simulink model "DA40_Flight_Model"  (R2023a)
settings: Solver=FixedStepAuto  StartTime=DCAM.startTime  StopTime=DCAM.endTime  FixedStep=DCAM.timeStep  RelTol=1e-3
undefined symbols (not defined in the file or in its folder): DCAM, Earth, WGS84
libraries: simulink x27, slpidlib x15, simulink_extras x6, sharedtransform x4, aerolibtransform2 x4, aerolibatmos2 x3, uavalgslib x2, aerolibwind2 x1
(part 1 of 6)
settings Model: Creator=izc0018  LastModifiedBy=noahm
settings DebuggingCC: AlgebraicLoopMsg=none  UnconnectedInputMsg=warning  UnconnectedOutputMsg=warning  UnconnectedLineMsg=warning
settings HardwareCC: ProdBitPerLong=64  ProdLargestAtomicFloat=None  ProdHWDeviceType=AMD->Athlon 64
settings ModelReferenceCC: EnableRefExpFcnMdlSchedulingChecks=on  ModelReferenceMinAlgLoopOccurrences=on
settings RTWCC: DLArmComputeVersion=19.05

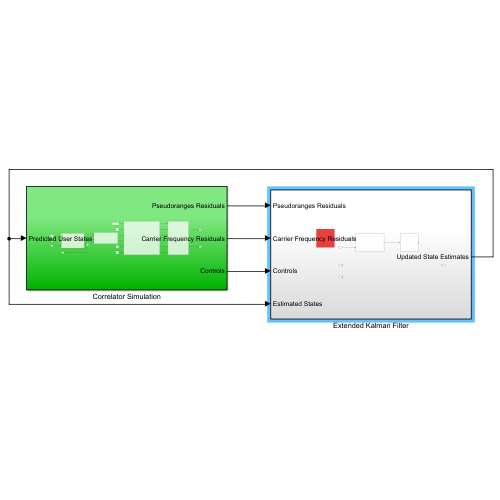
[thumbnail: Simulink's stored preview of the top-level diagram]
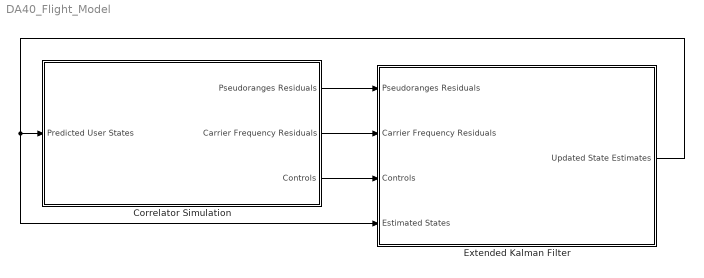
== system DA40_Flight_Model ==
  Correlator Simulation : Subsystem
  Extended Kalman Filter : Subsystem
  wires:
  Extended Kalman Filter/1(Updated State Estimates) -> Extended Kalman Filter/4(Estimated States), Correlator Simulation/1(Predicted User States)
  Correlator Simulation/1(Pseudoranges Residuals) -> Extended Kalman Filter/1(Pseudoranges Residuals)
  Correlator Simulation/2(Carrier Frequency Residuals) -> Extended Kalman Filter/2(Carrier Frequency Residuals)
  Correlator Simulation/3(Controls) -> Extended Kalman Filter/3(Controls)

== system DA40_Flight_Model/Correlator Simulation ==
  Predicted User States : Inport
  Band-Limited White Noise : simulink/Sources/Band-Limited White Noise  Cov=1  Ts=1/50  seed=DCAM.currentSeed
  Clock : Clock
  Constant : Constant  Value=0.5
  Constant1 : Constant  Value=1/50
  Constant2 : Constant  Value=10^(45/10)
  Constant3 : Constant  Value=0
  MATLAB Function : MATLAB Function  TreatAsAtomicUnit=on
  MATLAB Function1 : MATLAB Function  TreatAsAtomicUnit=on
  Subsystem : Subsystem
  Subsystem1 : Subsystem
  Terminator : Terminator
  Pseudoranges Residuals : Outport
  Carrier Frequency Residuals : Outport  Port=2
  Controls : Outport  Port=3
  wires:
  Constant/1 -> MATLAB Function/5(offset)
  Constant1/1 -> MATLAB Function/2(pdiTime)
  Band-Limited White Noise/1 -> MATLAB Function/6(whiteNoise)
  Constant2/1 -> MATLAB Function/1(cno)
  Subsystem/1(carrFreqError) -> MATLAB Function/3(carrFreqError)
  Subsystem/2(codeFreqError) -> MATLAB Function/4(codePhaseError)
  Constant3/1 -> Subsystem1/1(time)
  Clock/1 -> Subsystem1/2(time1)
  Subsystem1/1(MeasuredCarrierFrequency) -> Subsystem/1(measuredCarrierFrequency)
  Subsystem1/2(MeasuredCodeFrequency) -> Subsystem/2(measuredCodeFrequency)
  Subsystem1/6(Controls) -> Controls/1
  Predicted User States/1 -> Subsystem1/3(Predicted User States)
  Subsystem1/4(EstimatedCodeFrequency) -> Subsystem/4(estimatedCodeFrequency)
  Subsystem1/3(EstimatedCarrierFrequency) -> Subsystem/3(estimatedCarrierFrequency)
  MATLAB Function/6(QL) -> MATLAB Function1/6(QL)
  MATLAB Function/5(IL) -> MATLAB Function1/5(IL)
  MATLAB Function/4(QP) -> MATLAB Function1/4(QP)
  MATLAB Function/3(IP) -> MATLAB Function1/3(IP)
  MATLAB Function/2(QE) -> MATLAB Function1/2(QE)
  MATLAB Function/1(IE) -> MATLAB Function1/1(IE)
  MATLAB Function1/2(codeFreqResiduals) -> Pseudoranges Residuals/1
  MATLAB Function1/1(carrierFreqResiduals) -> Carrier Frequency Residuals/1
  Subsystem1/5(Measured Pseudoranges) -> Terminator/1

== system DA40_Flight_Model/Extended Kalman Filter ==
  Pseudoranges Residuals : Inport
  Carrier Frequency Residuals : Inport  Port=2
  Controls : Inport  Port=3
  Estimated States : Inport  Port=4
  Body To ECEF : Subsystem
  ECEF to BODY : Subsystem
  Noise Model : Subsystem
  Updated State Estimates : Outport
  wires:
  Noise Model/1(Predicted States) -> Body To ECEF/1(Predicted States)
  Controls/1 -> Noise Model/2(Controls)
  ECEF to BODY/1(ECEF States) -> Noise Model/1(Estimated States)
  Estimated States/1 -> ECEF to BODY/1(Estimated States)

== system DA40_Flight_Model/Correlator Simulation/Subsystem ==
  measuredCarrierFrequency : Inport
  measuredCodeFrequency : Inport  Port=2
  estimatedCarrierFrequency : Inport  Port=3
  estimatedCodeFrequency : Inport  Port=4
  MATLAB Function1 : MATLAB Function  TreatAsAtomicUnit=on
  MATLAB Function2 : MATLAB Function  TreatAsAtomicUnit=on
  carrFreqError : Outport
  codeFreqError : Outport  Port=2
  wires:
  measuredCarrierFrequency/1 -> MATLAB Function1/1(measuredCarrierFrequency)
  estimatedCarrierFrequency/1 -> MATLAB Function1/2(estimatedCarrierFrequency)
  MATLAB Function1/1(carrFreqError) -> carrFreqError/1
  estimatedCodeFrequency/1 -> MATLAB Function2/2(estimatedCodeFrequency)
  MATLAB Function2/1(codeFreqError) -> codeFreqError/1
  measuredCodeFrequency/1 -> MATLAB Function2/1(measuredCodeFrequency)

== system DA40_Flight_Model/Correlator Simulation/Subsystem1 ==
  time : Inport
  time1 : Inport  Port=2
  Predicted User States : Inport  Port=3
  Generating GPS and Satellite Measurements : Subsystem
  Generating GPS and Satellite Measurements1 : Subsystem
  Subsystem2 : Subsystem
  MeasuredCarrierFrequency : Outport
  MeasuredCodeFrequency : Outport  Port=2
  EstimatedCarrierFrequency : Outport  Port=3
  EstimatedCodeFrequency : Outport  Port=4
  Measured Pseudoranges : Outport  Port=5
  Controls : Outport  Port=6
  wires:
  Generating GPS and Satellite Measurements/2(Satellite States) -> Subsystem2/4(Satellite States)
  Subsystem2/1(MeasuredCarrierFrequency) -> MeasuredCarrierFrequency/1
  Generating GPS and Satellite Measurements/3(Controls) -> Controls/1
  Generating GPS and Satellite Measurements/1(GPS User States) -> Subsystem2/3(GPS User States)
  Generating GPS and Satellite Measurements1/1(GPS User States) -> Subsystem2/1(Initial GPS User States)
  Generating GPS and Satellite Measurements1/2(Satellite States) -> Subsystem2/2(Initial Satellite States)
  Subsystem2/2(MeasuredCodeFrequency) -> MeasuredCodeFrequency/1
  time1/1 -> Generating GPS and Satellite Measurements/1(time)
  time/1 -> Generating GPS and Satellite Measurements1/1(time)
  Subsystem2/3(Measured Pseudoranges) -> Measured Pseudoranges/1
  Predicted User States/1 -> Subsystem2/5(Predicted User States)
  Subsystem2/4(EstimatedCarrierFrequency) -> EstimatedCarrierFrequency/1
  Subsystem2/5(EstimatedCodeFrequency) -> EstimatedCodeFrequency/1

== system DA40_Flight_Model/Extended Kalman Filter/Body To ECEF ==
  Predicted States : Inport
  Bus Creator : BusCreator  Inputs=8
  Bus Selector : BusSelector  OutputSignals=psi,theta,phi
  Bus Selector1 : BusSelector  OutputSignals=x,y,z
  Bus Selector2 : BusSelector  OutputSignals=x,y,z,u,v,w
  Constant : Constant  Value=0
  Constant1 : Constant  Value=89.0
  Constant2 : Constant  Value=0
  Direction Cosine Matrix ECEF to NED : aerolibtransform2/Direction Cosine Matrix ECEF to NED
  Flat Earth to LLA : aerolibtransform2/Flat Earth to LLA  units=Metric (MKS)  ptype=Earth (WGS84)  F=1/298.257223563  R=6378137  refPosPort=off  LL0=DCAM.FVDM.refLL  psi=0
  MATLAB Function : MATLAB Function  TreatAsAtomicUnit=on
  MATLAB Function1 : MATLAB Function  TreatAsAtomicUnit=on
  Rotation Angles to Direction Cosine Matrix : sharedtransform/Rotation Angles to Direction Cosine Matrix  rotationOrder=ZYX  aMode=aMode
  Terminator : Terminator
  Transpose : Math  Operator=transpose
  Vector Concatenate{,1..3} (4 alike) : Concatenate  NumInputs=3
  ECEF States : Outport
  wires:
  Predicted States/1 -> Bus Selector2/1, Bus Selector1/1, Bus Selector/1
  Bus Selector/1 -> Vector Concatenate/1  "<psi>"
  Bus Selector/2 -> Vector Concatenate/2  "<theta>"
  Bus Selector/3 -> Vector Concatenate/3  "<phi>"
  Vector Concatenate/1 -> Rotation Angles to Direction Cosine Matrix/1
  Flat Earth to LLA/1 -> Direction Cosine Matrix ECEF to NED/1
  Flat Earth to LLA/2 -> Terminator/1
  Constant/1 -> Flat Earth to LLA/2
  Vector Concatenate1/1 -> Flat Earth to LLA/1
  Bus Selector1/1 -> Vector Concatenate1/1  "<x>"
  Bus Selector1/2 -> Vector Concatenate1/2  "<y>"
  Bus Selector1/3 -> Vector Concatenate1/3  "<z>"
  Direction Cosine Matrix ECEF to NED/1 -> Transpose/1
  Transpose/1 -> MATLAB Function/2(DCM_NE)  "NED TO ECEF"
  Rotation Angles to Direction Cosine Matrix/1 -> MATLAB Function/1(DCM_BN)  "BODY TO NED"
  MATLAB Function/1(DCM_BE) -> MATLAB Function1/5(DCM_BE)
  MATLAB Function1/8(clkBias) -> Bus Creator/8
  MATLAB Function1/7(clk) -> Bus Creator/7
  MATLAB Function1/6(w) -> Bus Creator/6
  MATLAB Function1/5(v) -> Bus Creator/5
  MATLAB Function1/4(u) -> Bus Creator/4
  MATLAB Function1/3(z) -> Bus Creator/3
  MATLAB Function1/2(y) -> Bus Creator/2
  MATLAB Function1/1(x) -> Bus Creator/1
  Bus Creator/1 -> ECEF States/1
  Constant1/1 -> MATLAB Function1/4("clkBias ")
  Constant2/1 -> MATLAB Function1/3("clk ")
  Vector Concatenate2/1 -> MATLAB Function1/1(pos)
  Vector Concatenate3/1 -> MATLAB Function1/2(vel)
  Bus Selector2/1 -> Vector Concatenate2/1  "<x>"
  Bus Selector2/2 -> Vector Concatenate2/2  "<y>"
  Bus Selector2/3 -> Vector Concatenate2/3  "<z>"
  Bus Selector2/4 -> Vector Concatenate3/1  "<u>"
  Bus Selector2/5 -> Vector Concatenate3/2  "<v>"
  Bus Selector2/6 -> Vector Concatenate3/3  "<w>"

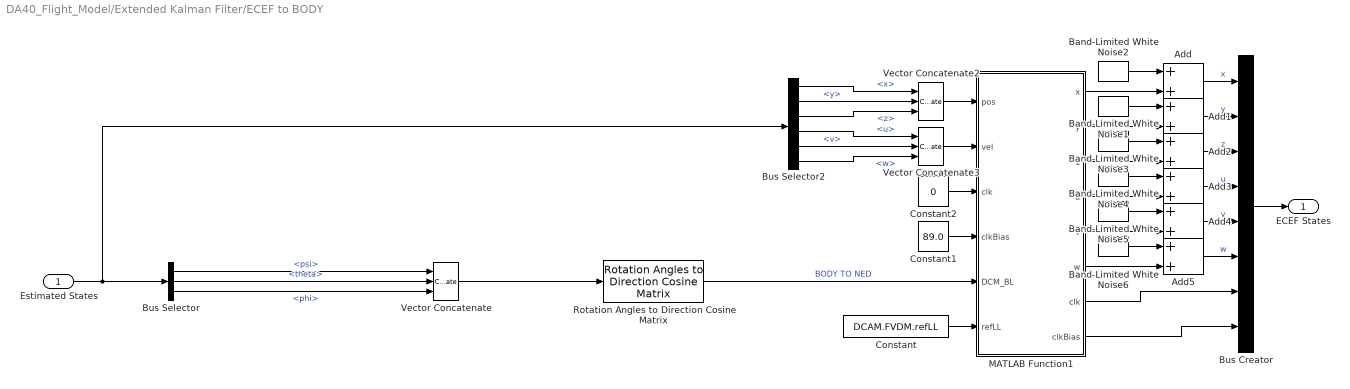
== system DA40_Flight_Model/Extended Kalman Filter/ECEF to BODY ==
  Estimated States : Inport
  Add{,1..5} (6 alike) : Sum
  Band-Limited White Noise1 : simulink/Sources/Band-Limited White Noise  Cov=1.5  Ts=1/50  seed=[23341]
  Band-Limited White Noise2 : simulink/Sources/Band-Limited White Noise  Cov=1.5  Ts=1/50  seed=[23341]
  Band-Limited White Noise3 : simulink/Sources/Band-Limited White Noise  Cov=3  Ts=1/50  seed=[23341]
  Band-Limited White Noise4 : simulink/Sources/Band-Limited White Noise  Cov=0.15  Ts=1/50  seed=[23341]
  Band-Limited White Noise5 : simulink/Sources/Band-Limited White Noise  Cov=0.15  Ts=1/50  seed=[23341]
  Band-Limited White Noise6 : simulink/Sources/Band-Limited White Noise  Cov=0.3  Ts=1/50  seed=[23341]
  Bus Creator : BusCreator  Inputs=8
  Bus Selector : BusSelector  OutputSignals=psi,theta,phi
  Bus Selector2 : BusSelector  OutputSignals=x,y,z,u,v,w
  Constant : Constant  Value=DCAM.FVDM.refLL
  Constant1 : Constant  Value=89.0
  Constant2 : Constant  Value=0
  MATLAB Function1 : MATLAB Function  TreatAsAtomicUnit=on
  Rotation Angles to Direction Cosine Matrix : sharedtransform/Rotation Angles to Direction Cosine Matrix  rotationOrder=ZYX  aMode=aMode
  Vector Concatenate : Concatenate  NumInputs=3
  Vector Concatenate2 : Concatenate  NumInputs=3
  Vector Concatenate3 : Concatenate  NumInputs=3
  ECEF States : Outport
  wires:
  Estimated States/1 -> Bus Selector2/1, Bus Selector/1
  Bus Selector/1 -> Vector Concatenate/1  "<psi>"
  Bus Selector/2 -> Vector Concatenate/2  "<theta>"
  Bus Selector/3 -> Vector Concatenate/3  "<phi>"
  Vector Concatenate/1 -> Rotation Angles to Direction Cosine Matrix/1
  Rotation Angles to Direction Cosine Matrix/1 -> MATLAB Function1/5(DCM_BL)  "BODY TO NED"
  MATLAB Function1/8(clkBias) -> Bus Creator/8
  MATLAB Function1/7(clk) -> Bus Creator/7
  Bus Creator/1 -> ECEF States/1
  Constant1/1 -> MATLAB Function1/4("clkBias ")
  Constant2/1 -> MATLAB Function1/3("clk ")
  Vector Concatenate2/1 -> MATLAB Function1/1(pos)
  Vector Concatenate3/1 -> MATLAB Function1/2(vel)
  Bus Selector2/1 -> Vector Concatenate2/1  "<x>"
  Bus Selector2/2 -> Vector Concatenate2/2  "<y>"
  Bus Selector2/3 -> Vector Concatenate2/3  "<z>"
  Bus Selector2/4 -> Vector Concatenate3/1  "<u>"
  Bus Selector2/5 -> Vector Concatenate3/2  "<v>"
  Bus Selector2/6 -> Vector Concatenate3/3  "<w>"
  Add/1 -> Bus Creator/1  "x"
  MATLAB Function1/1(x) -> Add/2
  Add1/1 -> Bus Creator/2  "y"
  Add2/1 -> Bus Creator/3  "z"
  Add3/1 -> Bus Creator/4  "u"
  Add4/1 -> Bus Creator/5  "v"
  Add5/1 -> Bus Creator/6  "w"
  Band-Limited White Noise1/1 -> Add1/1
  Band-Limited White Noise2/1 -> Add/1
  Band-Limited White Noise3/1 -> Add2/1
  Band-Limited White Noise4/1 -> Add3/1
  Band-Limited White Noise5/1 -> Add4/1
  Band-Limited White Noise6/1 -> Add5/1
  MATLAB Function1/2(y) -> Add1/2
  MATLAB Function1/3(z) -> Add2/2
  MATLAB Function1/4(u) -> Add3/2
  MATLAB Function1/5(v) -> Add4/2
  MATLAB Function1/6(w) -> Add5/2
  Constant/1 -> MATLAB Function1/6(refLL)

== system DA40_Flight_Model/Extended Kalman Filter/Noise Model ==
  Estimated States : Inport
  Controls : Inport  Port=2
  Band-Limited White Noise1 : simulink/Sources/Band-Limited White Noise  Cov=DCAM.FVDM.wind.direction  Ts=DCAM.FVDM.wind.directionTS  seed=DCAM.currentSeed
  Band-Limited White Noise3 : simulink/Sources/Band-Limited White Noise  Cov=DCAM.FVDM.wind.velocity  Ts=DCAM.FVDM.wind.velocityTS  seed=DCAM.currentSeed
  Environment : Subsystem
  Navigation : Subsystem
  Predicted States : Outport
  wires:
  Environment/1(Atmos) -> Navigation/1(Atmosphere)
  Navigation/1(States) -> Predicted States/1
  Band-Limited White Noise3/1 -> Environment/2(Wind Velocity)
  Controls/1 -> Navigation/2(Controls)
  Band-Limited White Noise1/1 -> Environment/3(Wind Direction)
  Estimated States/1 -> Environment/1(States)

== system DA40_Flight_Model/Correlator Simulation/Subsystem1/Generating GPS and Satellite Measurements ==
  time : Inport
  Body To ECEF : Subsystem
  Calculate Satellite Positions : Subsystem
  Truth Model : Subsystem
  GPS User States : Outport
  Satellite States : Outport  Port=2
  Controls : Outport  Port=3
  wires:
  time/1 -> Calculate Satellite Positions/1(time)
  Calculate Satellite Positions/1(Satellite States) -> Satellite States/1
  Truth Model/2(Truth States) -> Body To ECEF/1(Predicted States)
  Body To ECEF/1(ECEF States) -> GPS User States/1
  Truth Model/1(Controls) -> Controls/1

== system DA40_Flight_Model/Correlator Simulation/Subsystem1/Generating GPS and Satellite Measurements1 ==
  time : Inport
  Body To ECEF : Subsystem
  Calculate Satellite Positions : Subsystem
  Truth Model : Subsystem
  GPS User States : Outport
  Satellite States : Outport  Port=2
  wires:
  time/1 -> Calculate Satellite Positions/1(time)
  Calculate Satellite Positions/1(Satellite States) -> Satellite States/1
  Truth Model/1(Truth States) -> Body To ECEF/1(Predicted States)
  Body To ECEF/1(ECEF States) -> GPS User States/1

== system DA40_Flight_Model/Correlator Simulation/Subsystem1/Subsystem2 ==
  Initial GPS User States : Inport
  Initial Satellite States : Inport  Port=2
  GPS User States : Inport  Port=3
  Satellite States : Inport  Port=4
  Predicted User States : Inport  Port=5
  Generating PSR/Carrier Frequency Measurements : Subsystem
  Generating PSR/Carrier Frequency Measurements1 : Subsystem
  Generating PSR/Carrier Frequency Measurements2 : Subsystem
  Subsystem1 : Subsystem
  Subsystem2 : Subsystem
  Subsystem3 : Subsystem
  Subsystem4 : Subsystem
  MeasuredCarrierFrequency : Outport
  MeasuredCodeFrequency : Outport  Port=2
  Measured Pseudoranges : Outport  Port=3
  EstimatedCarrierFrequency : Outport  Port=4
  EstimatedCodeFrequency : Outport  Port=5
  wires:
  Subsystem3/1(sampleVector) -> Subsystem1/1(sampleVector)
  Generating PSR/Carrier Frequency Measurements/2(Measured Doppler) -> Subsystem3/5(doppler)
  Subsystem3/2(carrierChangePerSample) -> Subsystem1/2(carrierChangePerSample)
  Generating PSR/Carrier Frequency Measurements/1(Measured Carrier Frequencies) -> Subsystem3/4(measuredCarrierFrequency)
  Generating PSR/Carrier Frequency Measurements/3(Measured SV Clock Bias) -> Subsystem3/6(svClockBias)
  Subsystem3/3(CarrierFrequency) -> Subsystem1/3(measuredCarrierFrequency)
  GPS User States/1 -> Generating PSR/Carrier Frequency Measurements/1(GPS User States)
  Subsystem3/4(codeChangePerSample) -> Subsystem1/4(codeChangePerSample)
  Subsystem1/1(MeasuredCarrierFrequency) -> MeasuredCarrierFrequency/1
  Subsystem3/5(initialCodePhase) -> Subsystem1/5(initialCodePhase)
  Generating PSR/Carrier Frequency Measurements/4(Measured Pseudoranges) -> Measured Pseudoranges/1
  Satellite States/1 -> Generating PSR/Carrier Frequency Measurements2/1(Satellite States), Generating PSR/Carrier Frequency Measurements/2(Satellite States)
  Subsystem1/2(MeasuredCodeFrequency) -> MeasuredCodeFrequency/1
  Generating PSR/Carrier Frequency Measurements1/4(Initial SV Clock Bias) -> Subsystem3/3(initialSVClockBias)
  Generating PSR/Carrier Frequency Measurements1/3(Initial Doppler) -> Subsystem3/2(initialDoppler)
  Generating PSR/Carrier Frequency Measurements1/2(Initial Carrier Frequencies) -> Subsystem2/1(initialCarrierFrequency), Subsystem3/1(initialCarrierFrequency), Subsystem2/2(initialDoppler), Subsystem2/3(initialSVClockBias)
  Initial Satellite States/1 -> Generating PSR/Carrier Frequency Measurements1/2(Satellite States)
  Initial GPS User States/1 -> Generating PSR/Carrier Frequency Measurements1/1(GPS User States)
  Predicted User States/1 -> Generating PSR/Carrier Frequency Measurements2/2(Predicted User States)
  Generating PSR/Carrier Frequency Measurements2/1(Estimated Carrier Frequencies) -> Subsystem2/4(estimatedCarrierFrequency)
  Generating PSR/Carrier Frequency Measurements2/2(Estimated Doppler) -> Subsystem2/5(doppler)
  Generating PSR/Carrier Frequency Measurements2/3(Estimated SV Clock Bias) -> Subsystem2/6(svClockBias)
  Subsystem2/1(sampleVector) -> Subsystem4/1(sampleVector)
  Subsystem2/2(carrierChangePerSample) -> Subsystem4/2(carrierChangePerSample)
  Subsystem2/3(CarrierFrequency) -> Subsystem4/3(measuredCarrierFrequency)
  Subsystem2/4(codeChangePerSample) -> Subsystem4/4(codeChangePerSample)
  Subsystem2/5(initialCodePhase) -> Subsystem4/5(initialCodePhase)
  Subsystem4/1(EstimatedCarrierFrequency) -> EstimatedCarrierFrequency/1
  Subsystem4/2(EstimatedCodeFrequency) -> EstimatedCodeFrequency/1

== system DA40_Flight_Model/Extended Kalman Filter/Noise Model/Environment ==
  States : Inport
  Wind Velocity : Inport  Port=2
  Wind Direction : Inport  Port=3
  Bus Creator : BusCreator  Inputs=5
  Constant6 : Constant  Value=[3 2 1]
  Gain : Gain  Gain=180/pi
  Gain1 : Gain  Gain=-1
  Horizontal Wind Model : aerolibwind2/Horizontal Wind Model  units=Metric (MKS)  Vw_source=External  Vwind=0  W_source=External  Wdeg=0
  ISA Atmosphere Model : aerolibatmos2/ISA Atmosphere Model  custom=off  g=9.80665  gamma=1.4  R=287.0531  L=0.0065  h_trop=11000  h_strat=20000  rho0=1.225  P0=101325  T0=288.15  h0=0
  MATLAB Function7 : MATLAB Function  TreatAsAtomicUnit=on
  Selector : Selector  InputPortWidth=12  IndexOptions=Index vector (dialog)  Indices=[10 11 12]  OutputSizes=1
  Selector1 : Selector  InputPortWidth=12  IndexOptions=Index vector (dialog)  Indices=[9]  OutputSizes=1
  Atmos : Outport
  wires:
  MATLAB Function7/1(DCM) -> Horizontal Wind Model/1
  States/1 -> Selector/1, Selector1/1
  Selector1/1 -> Gain1/1
  ISA Atmosphere Model/2 -> Bus Creator/2  "Speed of Sound"
  ISA Atmosphere Model/3 -> Bus Creator/3  "Pressure"
  Bus Creator/1 -> Atmos/1
  Selector/1 -> Gain/1
  ISA Atmosphere Model/1 -> Bus Creator/1  "Temperature"
  Gain/1 -> MATLAB Function7/1(RotAngles)
  ISA Atmosphere Model/4 -> Bus Creator/4  "Density"
  Constant6/1 -> MATLAB Function7/2(RotSequence)
  Horizontal Wind Model/1 -> Bus Creator/5  "Wind Vector"
  Gain1/1 -> ISA Atmosphere Model/1
  Wind Velocity/1 -> Horizontal Wind Model/2
  Wind Direction/1 -> Horizontal Wind Model/3

== system DA40_Flight_Model/Extended Kalman Filter/Noise Model/Navigation ==
  Atmosphere : Inport
  Controls : Inport  Port=2
  Constant1 : Constant  Value=DCAM.FVDM.Vehicle.MassProp.Mass
  DA-40 Equations of Motion : Subsystem
  Flight Mechanics and Systems Models : Subsystem
  States : Outport
  wires:
  Flight Mechanics and Systems Models/1(Fb) -> DA-40 Equations of Motion/1(Fb [lb])
  Flight Mechanics and Systems Models/2(Mb) -> DA-40 Equations of Motion/2(Mb [lb-ft])
  Controls/1 -> Flight Mechanics and Systems Models/2(Control Commands)
  Atmosphere/1 -> Flight Mechanics and Systems Models/1(Atmosphere)
  Constant1/1 -> DA-40 Equations of Motion/3(Mass Properties)
  DA-40 Equations of Motion/1(States) -> States/1, Flight Mechanics and Systems Models/3(States)

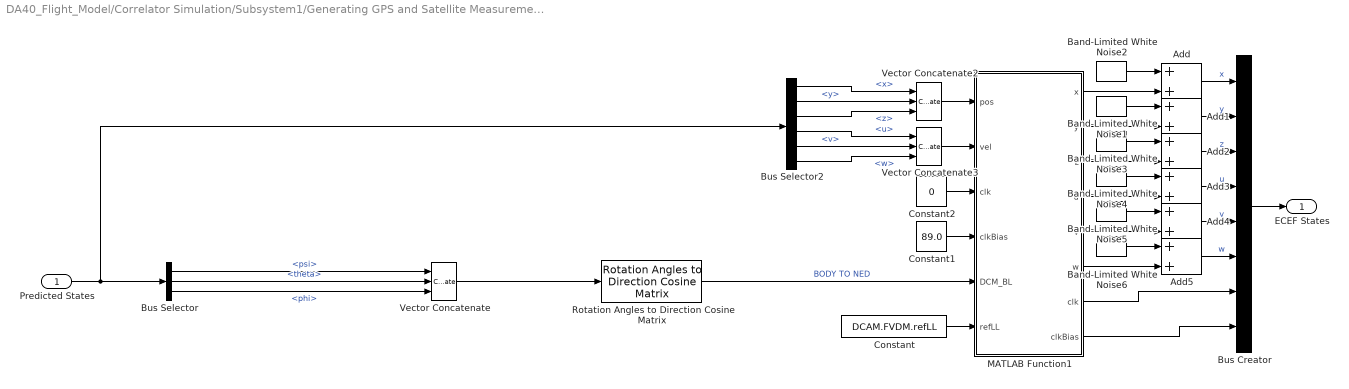
== system DA40_Flight_Model/Correlator Simulation/Subsystem1/Generating GPS and Satellite Measurements/Body To ECEF ==
  Predicted States : Inport
  Add{,1..5} (6 alike) : Sum
  Band-Limited White Noise1 : simulink/Sources/Band-Limited White Noise  Cov=1.5  Ts=1/50  seed=[23341]
  Band-Limited White Noise2 : simulink/Sources/Band-Limited White Noise  Cov=1.5  Ts=1/50  seed=[23341]
  Band-Limited White Noise3 : simulink/Sources/Band-Limited White Noise  Cov=3  Ts=1/50  seed=[23341]
  Band-Limited White Noise4 : simulink/Sources/Band-Limited White Noise  Cov=0.15  Ts=1/50  seed=[23341]
  Band-Limited White Noise5 : simulink/Sources/Band-Limited White Noise  Cov=0.15  Ts=1/50  seed=[23341]
  Band-Limited White Noise6 : simulink/Sources/Band-Limited White Noise  Cov=0.3  Ts=1/50  seed=[23341]
  Bus Creator : BusCreator  Inputs=8
  Bus Selector : BusSelector  OutputSignals=psi,theta,phi
  Bus Selector2 : BusSelector  OutputSignals=x,y,z,u,v,w
  Constant : Constant  Value=DCAM.FVDM.refLL
  Constant1 : Constant  Value=89.0
  Constant2 : Constant  Value=0
  MATLAB Function1 : MATLAB Function  TreatAsAtomicUnit=on
  Rotation Angles to Direction Cosine Matrix : sharedtransform/Rotation Angles to Direction Cosine Matrix  rotationOrder=ZYX  aMode=aMode
  Vector Concatenate : Concatenate  NumInputs=3
  Vector Concatenate2 : Concatenate  NumInputs=3
  Vector Concatenate3 : Concatenate  NumInputs=3
  ECEF States : Outport
  wires:
  Predicted States/1 -> Bus Selector2/1, Bus Selector/1
  Bus Selector/1 -> Vector Concatenate/1  "<psi>"
  Bus Selector/2 -> Vector Concatenate/2  "<theta>"
  Bus Selector/3 -> Vector Concatenate/3  "<phi>"
  Vector Concatenate/1 -> Rotation Angles to Direction Cosine Matrix/1
  Rotation Angles to Direction Cosine Matrix/1 -> MATLAB Function1/5(DCM_BL)  "BODY TO NED"
  MATLAB Function1/8(clkBias) -> Bus Creator/8
  MATLAB Function1/7(clk) -> Bus Creator/7
  Bus Creator/1 -> ECEF States/1
  Constant1/1 -> MATLAB Function1/4("clkBias ")
  Constant2/1 -> MATLAB Function1/3("clk ")
  Vector Concatenate2/1 -> MATLAB Function1/1(pos)
  Vector Concatenate3/1 -> MATLAB Function1/2(vel)
  Bus Selector2/1 -> Vector Concatenate2/1  "<x>"
  Bus Selector2/2 -> Vector Concatenate2/2  "<y>"
  Bus Selector2/3 -> Vector Concatenate2/3  "<z>"
  Bus Selector2/4 -> Vector Concatenate3/1  "<u>"
  Bus Selector2/5 -> Vector Concatenate3/2  "<v>"
  Bus Selector2/6 -> Vector Concatenate3/3  "<w>"
  Add/1 -> Bus Creator/1  "x"
  MATLAB Function1/1(x) -> Add/2
  Add1/1 -> Bus Creator/2  "y"
  Add2/1 -> Bus Creator/3  "z"
  Add3/1 -> Bus Creator/4  "u"
  Add4/1 -> Bus Creator/5  "v"
  Add5/1 -> Bus Creator/6  "w"
  Band-Limited White Noise1/1 -> Add1/1
  Band-Limited White Noise2/1 -> Add/1
  Band-Limited White Noise3/1 -> Add2/1
  Band-Limited White Noise4/1 -> Add3/1
  Band-Limited White Noise5/1 -> Add4/1
  Band-Limited White Noise6/1 -> Add5/1
  MATLAB Function1/2(y) -> Add1/2
  MATLAB Function1/3(z) -> Add2/2
  MATLAB Function1/4(u) -> Add3/2
  MATLAB Function1/5(v) -> Add4/2
  MATLAB Function1/6(w) -> Add5/2
  Constant/1 -> MATLAB Function1/6(refLL)

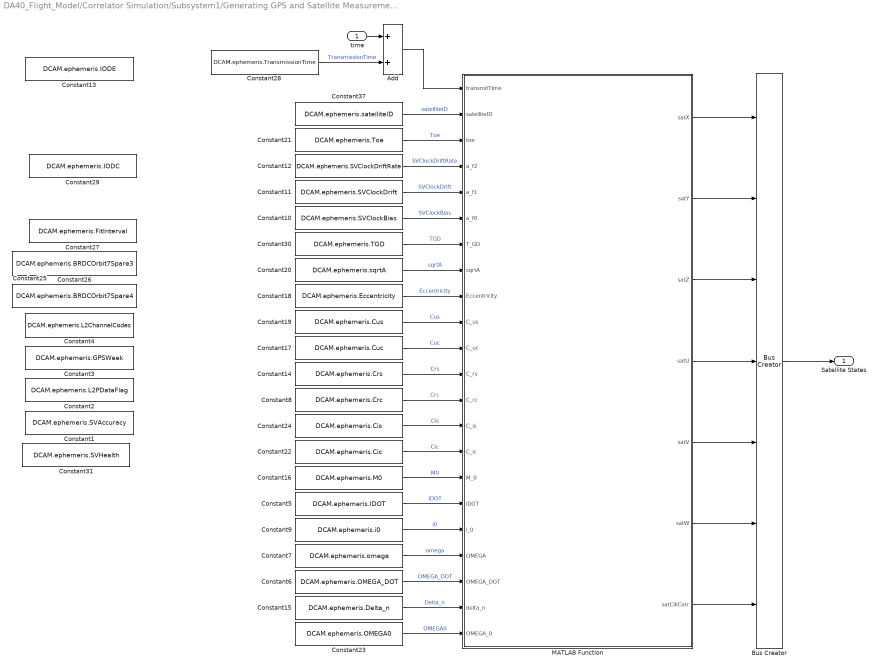
== system DA40_Flight_Model/Correlator Simulation/Subsystem1/Generating GPS and Satellite Measurements/Calculate Satellite Positions ==
  time : Inport
  Add : Sum
  Bus Creator : BusCreator  Inputs=7
  Constant1 : Constant  Value=DCAM.ephemeris.SVAccuracy
  Constant10 : Constant  Value=DCAM.ephemeris.SVClockBias
  Constant11 : Constant  Value=DCAM.ephemeris.SVClockDrift
  Constant12 : Constant  Value=DCAM.ephemeris.SVClockDriftRate
  Constant13 : Constant  Value=DCAM.ephemeris.IODE
  Constant14 : Constant  Value=DCAM.ephemeris.Crs
  Constant15 : Constant  Value=DCAM.ephemeris.Delta_n
  Constant16 : Constant  Value=DCAM.ephemeris.M0
  Constant17 : Constant  Value=DCAM.ephemeris.Cuc
  Constant18 : Constant  Value=DCAM.ephemeris.Eccentricity
  Constant19 : Constant  Value=DCAM.ephemeris.Cus
  Constant2 : Constant  Value=DCAM.ephemeris.L2PDataFlag
  Constant20 : Constant  Value=DCAM.ephemeris.sqrtA
  Constant21 : Constant  Value=DCAM.ephemeris.Toe
  Constant22 : Constant  Value=DCAM.ephemeris.Cic
  Constant23 : Constant  Value=DCAM.ephemeris.OMEGA0
  Constant24 : Constant  Value=DCAM.ephemeris.Cis
  Constant25 : Constant  Value=DCAM.ephemeris.BRDCOrbit7Spare4
  Constant26 : Constant  Value=DCAM.ephemeris.BRDCOrbit7Spare3
  Constant27 : Constant  Value=DCAM.ephemeris.FitInterval
  Constant28 : Constant  Value=DCAM.ephemeris.TransmissionTime
  Constant29 : Constant  Value=DCAM.ephemeris.IODC
  Constant3 : Constant  Value=DCAM.ephemeris.GPSWeek
  Constant30 : Constant  Value=DCAM.ephemeris.TGD
  Constant31 : Constant  Value=DCAM.ephemeris.SVHealth
  Constant37 : Constant  Value=DCAM.ephemeris.satelliteID
  Constant4 : Constant  Value=DCAM.ephemeris.L2ChannelCodes
  Constant5 : Constant  Value=DCAM.ephemeris.IDOT
  Constant6 : Constant  Value=DCAM.ephemeris.OMEGA_DOT
  Constant7 : Constant  Value=DCAM.ephemeris.omega
  Constant8 : Constant  Value=DCAM.ephemeris.Crc
  Constant9 : Constant  Value=DCAM.ephemeris.i0
  MATLAB Function : MATLAB Function  TreatAsAtomicUnit=on
  Satellite States : Outport
  wires:
  Bus Creator/1 -> Satellite States/1
  MATLAB Function/7(satClkCorr) -> Bus Creator/7
  MATLAB Function/6(satW) -> Bus Creator/6
  MATLAB Function/5(satV) -> Bus Creator/5
  MATLAB Function/4(satU) -> Bus Creator/4
  MATLAB Function/3(satZ) -> Bus Creator/3
  MATLAB Function/2(satY) -> Bus Creator/2
  MATLAB Function/1(satX) -> Bus Creator/1
  Constant37/1 -> MATLAB Function/2(satelliteID)  "satelliteID"
  Constant21/1 -> MATLAB Function/3(toe)  "Toe"
  Constant12/1 -> MATLAB Function/4(a_f2)  "SVClockDriftRate"
  Constant11/1 -> MATLAB Function/5(a_f1)  "SVClockDrift"
  Constant10/1 -> MATLAB Function/6(a_f0)  "SVClockBias"
  Constant30/1 -> MATLAB Function/7(T_GD)  "TGD"
  Constant20/1 -> MATLAB Function/8(sqrtA)  "sqrtA"
  Constant18/1 -> MATLAB Function/9(Eccentricity)  "Eccentricity"
  Constant19/1 -> MATLAB Function/10(C_us)  "Cus"
  Constant17/1 -> MATLAB Function/11(C_uc)  "Cuc"
  Constant8/1 -> MATLAB Function/13(C_rc)  "Crc"
  Constant14/1 -> MATLAB Function/12(C_rs)  "Crs"
  Constant24/1 -> MATLAB Function/14(C_is)  "Cis"
  Constant22/1 -> MATLAB Function/15(C_ic)  "Cic"
  Constant16/1 -> MATLAB Function/16(M_0)  "M0"
  Constant5/1 -> MATLAB Function/17(iDOT)  "IDOT"
  Constant9/1 -> MATLAB Function/18(i_0)  "i0"
  Constant7/1 -> MATLAB Function/19(OMEGA)  "omega"
  Constant6/1 -> MATLAB Function/20(OMEGA_DOT)  "OMEGA_DOT"
  Add/1 -> MATLAB Function/1(transmitTime)
  time/1 -> Add/1
  Constant28/1 -> Add/2  "TransmissionTime"
  Constant15/1 -> MATLAB Function/21(delta_n)  "Delta_n"
  Constant23/1 -> MATLAB Function/22(OMEGA_0)  "OMEGA0"

== system DA40_Flight_Model/Correlator Simulation/Subsystem1/Generating GPS and Satellite Measurements/Truth Model ==
  Control : Subsystem
  Environment : Subsystem
  Guidance : Subsystem
  Navigation1 : Subsystem
  Controls : Outport
  Truth States : Outport  Port=2
  wires:
  Control/1(Controls) -> Navigation1/2(Controls), Controls/1
  Guidance/1(Commands) -> Control/1(Commands)
  Guidance/2(States Out) -> Control/2(States)
  Guidance/3(Atmos) -> Control/3(Atmos)
  Environment/1(States Out) -> Guidance/1(States)
  Environment/2(Atmos) -> Guidance/2(Atmosphere)
  Control/3(LLA) -> Environment/2(LLA)
  Control/2(Atmosphere) -> Navigation1/1(Atmosphere)
  Navigation1/1(States) -> Truth States/1, Environment/1(States)

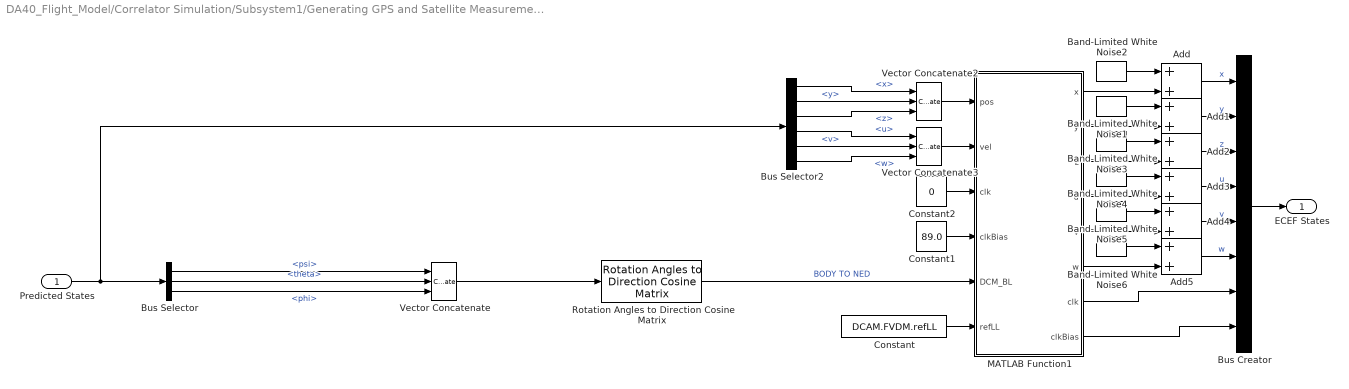
== system DA40_Flight_Model/Correlator Simulation/Subsystem1/Generating GPS and Satellite Measurements1/Body To ECEF ==
  Predicted States : Inport
  Add{,1..5} (6 alike) : Sum
  Band-Limited White Noise1 : simulink/Sources/Band-Limited White Noise  Cov=1.5  Ts=1/50  seed=[23341]
  Band-Limited White Noise2 : simulink/Sources/Band-Limited White Noise  Cov=1.5  Ts=1/50  seed=[23341]
  Band-Limited White Noise3 : simulink/Sources/Band-Limited White Noise  Cov=3  Ts=1/50  seed=[23341]
  Band-Limited White Noise4 : simulink/Sources/Band-Limited White Noise  Cov=0.15  Ts=1/50  seed=[23341]
  Band-Limited White Noise5 : simulink/Sources/Band-Limited White Noise  Cov=0.15  Ts=1/50  seed=[23341]
  Band-Limited White Noise6 : simulink/Sources/Band-Limited White Noise  Cov=0.3  Ts=1/50  seed=[23341]
  Bus Creator : BusCreator  Inputs=8
  Bus Selector : BusSelector  OutputSignals=psi,theta,phi
  Bus Selector2 : BusSelector  OutputSignals=x,y,z,u,v,w
  Constant : Constant  Value=DCAM.FVDM.refLL
  Constant1 : Constant  Value=89.0
  Constant2 : Constant  Value=0
  MATLAB Function1 : MATLAB Function  TreatAsAtomicUnit=on
  Rotation Angles to Direction Cosine Matrix : sharedtransform/Rotation Angles to Direction Cosine Matrix  rotationOrder=ZYX  aMode=aMode
  Vector Concatenate : Concatenate  NumInputs=3
  Vector Concatenate2 : Concatenate  NumInputs=3
  Vector Concatenate3 : Concatenate  NumInputs=3
  ECEF States : Outport
  wires:
  Predicted States/1 -> Bus Selector2/1, Bus Selector/1
  Bus Selector/1 -> Vector Concatenate/1  "<psi>"
  Bus Selector/2 -> Vector Concatenate/2  "<theta>"
  Bus Selector/3 -> Vector Concatenate/3  "<phi>"
  Vector Concatenate/1 -> Rotation Angles to Direction Cosine Matrix/1
  Rotation Angles to Direction Cosine Matrix/1 -> MATLAB Function1/5(DCM_BL)  "BODY TO NED"
  MATLAB Function1/8(clkBias) -> Bus Creator/8
  MATLAB Function1/7(clk) -> Bus Creator/7
  Bus Creator/1 -> ECEF States/1
  Constant1/1 -> MATLAB Function1/4("clkBias ")
  Constant2/1 -> MATLAB Function1/3("clk ")
  Vector Concatenate2/1 -> MATLAB Function1/1(pos)
  Vector Concatenate3/1 -> MATLAB Function1/2(vel)
  Bus Selector2/1 -> Vector Concatenate2/1  "<x>"
  Bus Selector2/2 -> Vector Concatenate2/2  "<y>"
  Bus Selector2/3 -> Vector Concatenate2/3  "<z>"
  Bus Selector2/4 -> Vector Concatenate3/1  "<u>"
  Bus Selector2/5 -> Vector Concatenate3/2  "<v>"
  Bus Selector2/6 -> Vector Concatenate3/3  "<w>"
  Add/1 -> Bus Creator/1  "x"
  MATLAB Function1/1(x) -> Add/2
  Add1/1 -> Bus Creator/2  "y"
  Add2/1 -> Bus Creator/3  "z"
  Add3/1 -> Bus Creator/4  "u"
  Add4/1 -> Bus Creator/5  "v"
  Add5/1 -> Bus Creator/6  "w"
  Band-Limited White Noise1/1 -> Add1/1
  Band-Limited White Noise2/1 -> Add/1
  Band-Limited White Noise3/1 -> Add2/1
  Band-Limited White Noise4/1 -> Add3/1
  Band-Limited White Noise5/1 -> Add4/1
  Band-Limited White Noise6/1 -> Add5/1
  MATLAB Function1/2(y) -> Add1/2
  MATLAB Function1/3(z) -> Add2/2
  MATLAB Function1/4(u) -> Add3/2
  MATLAB Function1/5(v) -> Add4/2
  MATLAB Function1/6(w) -> Add5/2
  Constant/1 -> MATLAB Function1/6(refLL)

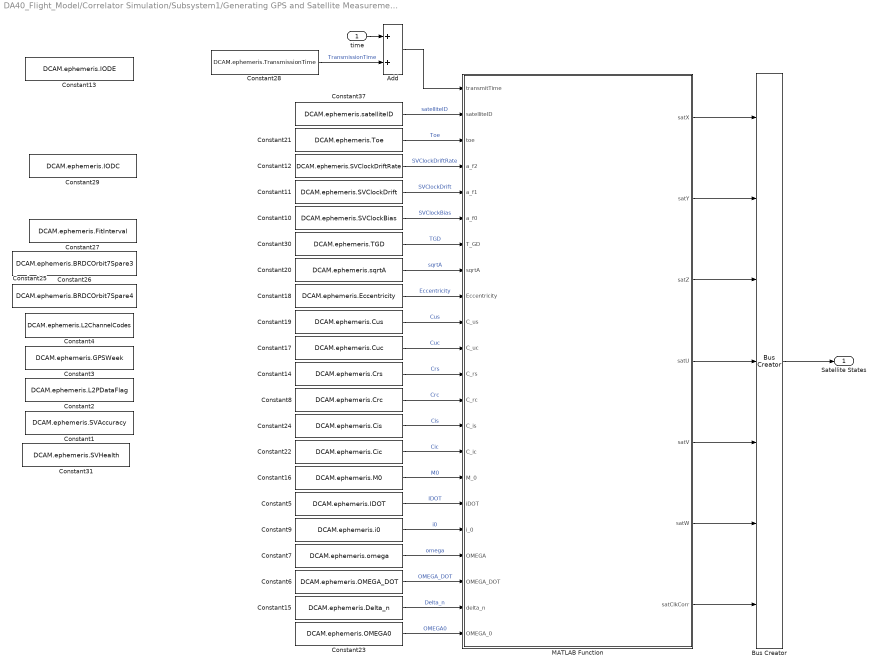
== system DA40_Flight_Model/Correlator Simulation/Subsystem1/Generating GPS and Satellite Measurements1/Calculate Satellite Positions ==
  time : Inport
  Add : Sum
  Bus Creator : BusCreator  Inputs=7
  Constant1 : Constant  Value=DCAM.ephemeris.SVAccuracy
  Constant10 : Constant  Value=DCAM.ephemeris.SVClockBias
  Constant11 : Constant  Value=DCAM.ephemeris.SVClockDrift
  Constant12 : Constant  Value=DCAM.ephemeris.SVClockDriftRate
  Constant13 : Constant  Value=DCAM.ephemeris.IODE
  Constant14 : Constant  Value=DCAM.ephemeris.Crs
  Constant15 : Constant  Value=DCAM.ephemeris.Delta_n
  Constant16 : Constant  Value=DCAM.ephemeris.M0
  Constant17 : Constant  Value=DCAM.ephemeris.Cuc
  Constant18 : Constant  Value=DCAM.ephemeris.Eccentricity
  Constant19 : Constant  Value=DCAM.ephemeris.Cus
  Constant2 : Constant  Value=DCAM.ephemeris.L2PDataFlag
  Constant20 : Constant  Value=DCAM.ephemeris.sqrtA
  Constant21 : Constant  Value=DCAM.ephemeris.Toe
  Constant22 : Constant  Value=DCAM.ephemeris.Cic
  Constant23 : Constant  Value=DCAM.ephemeris.OMEGA0
  Constant24 : Constant  Value=DCAM.ephemeris.Cis
  Constant25 : Constant  Value=DCAM.ephemeris.BRDCOrbit7Spare4
  Constant26 : Constant  Value=DCAM.ephemeris.BRDCOrbit7Spare3
  Constant27 : Constant  Value=DCAM.ephemeris.FitInterval
  Constant28 : Constant  Value=DCAM.ephemeris.TransmissionTime
  Constant29 : Constant  Value=DCAM.ephemeris.IODC
  Constant3 : Constant  Value=DCAM.ephemeris.GPSWeek
  Constant30 : Constant  Value=DCAM.ephemeris.TGD
  Constant31 : Constant  Value=DCAM.ephemeris.SVHealth
  Constant37 : Constant  Value=DCAM.ephemeris.satelliteID
  Constant4 : Constant  Value=DCAM.ephemeris.L2ChannelCodes
  Constant5 : Constant  Value=DCAM.ephemeris.IDOT
  Constant6 : Constant  Value=DCAM.ephemeris.OMEGA_DOT
  Constant7 : Constant  Value=DCAM.ephemeris.omega
  Constant8 : Constant  Value=DCAM.ephemeris.Crc
  Constant9 : Constant  Value=DCAM.ephemeris.i0
  MATLAB Function : MATLAB Function  TreatAsAtomicUnit=on
  Satellite States : Outport
  wires:
  Bus Creator/1 -> Satellite States/1
  MATLAB Function/7(satClkCorr) -> Bus Creator/7
  MATLAB Function/6(satW) -> Bus Creator/6
  MATLAB Function/5(satV) -> Bus Creator/5
  MATLAB Function/4(satU) -> Bus Creator/4
  MATLAB Function/3(satZ) -> Bus Creator/3
  MATLAB Function/2(satY) -> Bus Creator/2
  MATLAB Function/1(satX) -> Bus Creator/1
  Constant37/1 -> MATLAB Function/2(satelliteID)  "satelliteID"
  Constant21/1 -> MATLAB Function/3(toe)  "Toe"
  Constant12/1 -> MATLAB Function/4(a_f2)  "SVClockDriftRate"
  Constant11/1 -> MATLAB Function/5(a_f1)  "SVClockDrift"
  Constant10/1 -> MATLAB Function/6(a_f0)  "SVClockBias"
  Constant30/1 -> MATLAB Function/7(T_GD)  "TGD"
  Constant20/1 -> MATLAB Function/8(sqrtA)  "sqrtA"
  Constant18/1 -> MATLAB Function/9(Eccentricity)  "Eccentricity"
  Constant19/1 -> MATLAB Function/10(C_us)  "Cus"
  Constant17/1 -> MATLAB Function/11(C_uc)  "Cuc"
  Constant8/1 -> MATLAB Function/13(C_rc)  "Crc"
  Constant14/1 -> MATLAB Function/12(C_rs)  "Crs"
  Constant24/1 -> MATLAB Function/14(C_is)  "Cis"
  Constant22/1 -> MATLAB Function/15(C_ic)  "Cic"
  Constant16/1 -> MATLAB Function/16(M_0)  "M0"
  Constant5/1 -> MATLAB Function/17(iDOT)  "IDOT"
  Constant9/1 -> MATLAB Function/18(i_0)  "i0"
  Constant7/1 -> MATLAB Function/19(OMEGA)  "omega"
  Constant6/1 -> MATLAB Function/20(OMEGA_DOT)  "OMEGA_DOT"
  Add/1 -> MATLAB Function/1(transmitTime)
  time/1 -> Add/1
  Constant28/1 -> Add/2  "TransmissionTime"
  Constant15/1 -> MATLAB Function/21(delta_n)  "Delta_n"
  Constant23/1 -> MATLAB Function/22(OMEGA_0)  "OMEGA0"

== system DA40_Flight_Model/Correlator Simulation/Subsystem1/Generating GPS and Satellite Measurements1/Truth Model ==
  Control : Subsystem
  Environment : Subsystem
  Guidance : Subsystem
  Navigation1 : Subsystem
  Truth States : Outport
  wires:
  Control/1(Controls) -> Navigation1/2(Controls)
  Guidance/1(Commands) -> Control/1(Commands)
  Guidance/2(States Out) -> Control/2(States)
  Guidance/3(Atmos) -> Control/3(Atmos)
  Environment/1(States Out) -> Guidance/1(States)
  Environment/2(Atmos) -> Guidance/2(Atmosphere)
  Control/3(LLA) -> Environment/2(LLA)
  Control/2(Atmosphere) -> Navigation1/1(Atmosphere)
  Navigation1/1(States) -> Truth States/1, Environment/1(States)

== system DA40_Flight_Model/Correlator Simulation/Subsystem1/Subsystem2/Generating PSR//Carrier Frequency Measurements ==
  GPS User States : Inport
  Satellite States : Inport  Port=2
  Add : Sum  Inputs=+-
  Bus Selector : BusSelector  OutputSignals=x,y,z,clk
  Bus Selector1 : BusSelector  OutputSignals=satX,satY,satZ
  Bus Selector2 : BusSelector  OutputSignals=satU,satV,satW,satClkCorr
  Bus Selector3 : BusSelector  OutputSignals=u,v,w
  Constant : Constant  Value=4.092e6
  Constant1 : Constant  Value=0
  Constant2 : Constant  Value=1575.42e6
  Constant3 : Constant  Value=4.092e6
  MATLAB Function : MATLAB Function  TreatAsAtomicUnit=on
  MATLAB Function1 : MATLAB Function  TreatAsAtomicUnit=on
  Measured Carrier Frequencies : Outport
  Measured Doppler : Outport  Port=2
  Measured SV Clock Bias : Outport  Port=3
  Measured Pseudoranges : Outport  Port=4
  wires:
  MATLAB Function/1(pseudoranges) -> Measured Pseudoranges/1
  GPS User States/1 -> Bus Selector3/1, Bus Selector/1
  MATLAB Function1/1(carrFrequency) -> Add/1, Measured Carrier Frequencies/1
  Bus Selector/1 -> MATLAB Function/1(usrX)  "<x>"
  Bus Selector/2 -> MATLAB Function/2(usrY)  "<y>"
  Bus Selector/3 -> MATLAB Function/3(usrZ)  "<z>"
  Bus Selector/4 -> MATLAB Function/4(clk)  "<clk>"
  Satellite States/1 -> Bus Selector1/1, Bus Selector2/1
  Bus Selector1/3 -> MATLAB Function/7(satZ)  "<satZ>"
  Bus Selector1/2 -> MATLAB Function/6(satY)  "<satY>"
  Bus Selector1/1 -> MATLAB Function/5(satX)  "<satX>"
  MATLAB Function/2(unitVectors) -> MATLAB Function1/1(unitVectors)
  Bus Selector2/3 -> MATLAB Function1/7(satW)  "<satW>"
  Bus Selector2/2 -> MATLAB Function1/6(satV)  "<satV>"
  Bus Selector2/1 -> MATLAB Function1/5(satU)  "<satU>"
  Bus Selector3/3 -> MATLAB Function1/4(usrW)  "<w>"
  Bus Selector3/2 -> MATLAB Function1/3(usrV)  "<v>"
  Bus Selector3/1 -> MATLAB Function1/2(usrU)  "<u>"
  Add/1 -> Measured Doppler/1
  Constant/1 -> Add/2
  Constant1/1 -> MATLAB Function1/8(clkDrift)
  Constant2/1 -> MATLAB Function1/9(L1Freq)
  Constant3/1 -> MATLAB Function1/10(IFFreq)
  Bus Selector2/4 -> Measured SV Clock Bias/1  "<satClkCorr>"

== system DA40_Flight_Model/Correlator Simulation/Subsystem1/Subsystem2/Generating PSR//Carrier Frequency Measurements1 ==
  GPS User States : Inport
  Satellite States : Inport  Port=2
  Add : Sum  Inputs=+-
  Bus Selector : BusSelector  OutputSignals=x,y,z,clk
  Bus Selector1 : BusSelector  OutputSignals=satX,satY,satZ
  Bus Selector2 : BusSelector  OutputSignals=satU,satV,satW,satClkCorr
  Bus Selector3 : BusSelector  OutputSignals=u,v,w
  Constant : Constant  Value=4.092e6
  Constant1 : Constant  Value=0
  Constant2 : Constant  Value=1575.42e6
  Constant3 : Constant  Value=4.092e6
  MATLAB Function : MATLAB Function  TreatAsAtomicUnit=on
  MATLAB Function1 : MATLAB Function  TreatAsAtomicUnit=on
  Initial Pseudoranges : Outport
  Initial Carrier Frequencies : Outport  Port=2
  Initial Doppler : Outport  Port=3
  Initial SV Clock Bias : Outport  Port=4
  wires:
  MATLAB Function/1(pseudoranges) -> Initial Pseudoranges/1
  GPS User States/1 -> Bus Selector3/1, Bus Selector/1
  MATLAB Function1/1(carrFrequency) -> Add/1, Initial Carrier Frequencies/1
  Bus Selector/1 -> MATLAB Function/1(usrX)  "<x>"
  Bus Selector/2 -> MATLAB Function/2(usrY)  "<y>"
  Bus Selector/3 -> MATLAB Function/3(usrZ)  "<z>"
  Bus Selector/4 -> MATLAB Function/4(clk)  "<clk>"
  Satellite States/1 -> Bus Selector1/1, Bus Selector2/1
  Bus Selector1/3 -> MATLAB Function/7(satZ)  "<satZ>"
  Bus Selector1/2 -> MATLAB Function/6(satY)  "<satY>"
  Bus Selector1/1 -> MATLAB Function/5(satX)  "<satX>"
  MATLAB Function/2(unitVectors) -> MATLAB Function1/1(unitVectors)
  Bus Selector2/3 -> MATLAB Function1/7(satW)  "<satW>"
  Bus Selector2/2 -> MATLAB Function1/6(satV)  "<satV>"
  Bus Selector2/1 -> MATLAB Function1/5(satU)  "<satU>"
  Bus Selector3/3 -> MATLAB Function1/4(usrW)  "<w>"
  Bus Selector3/2 -> MATLAB Function1/3(usrV)  "<v>"
  Bus Selector3/1 -> MATLAB Function1/2(usrU)  "<u>"
  Add/1 -> Initial Doppler/1
  Constant/1 -> Add/2
  Constant1/1 -> MATLAB Function1/8(clkDrift)
  Constant2/1 -> MATLAB Function1/9(L1Freq)
  Constant3/1 -> MATLAB Function1/10(IFFreq)
  Bus Selector2/4 -> Initial SV Clock Bias/1  "<satClkCorr>"

== system DA40_Flight_Model/Correlator Simulation/Subsystem1/Subsystem2/Generating PSR//Carrier Frequency Measurements2 ==
  Satellite States : Inport
  Predicted User States : Inport  Port=2
  Add : Sum  Inputs=+-
  Bus Selector : BusSelector  OutputSignals=x,y,z,clk
  Bus Selector1 : BusSelector  OutputSignals=satX,satY,satZ
  Bus Selector2 : BusSelector  OutputSignals=satU,satV,satW,satClkCorr
  Bus Selector3 : BusSelector  OutputSignals=u,v,w
  Constant : Constant  Value=4.092e6
  Constant1 : Constant  Value=0
  Constant2 : Constant  Value=1575.42e6
  Constant3 : Constant  Value=4.092e6
  MATLAB Function : MATLAB Function  TreatAsAtomicUnit=on
  MATLAB Function1 : MATLAB Function  TreatAsAtomicUnit=on
  Estimated Carrier Frequencies : Outport
  Estimated Doppler : Outport  Port=2
  Estimated SV Clock Bias : Outport  Port=3
  Estimated Pseudoranges : Outport  Port=4
  wires:
  MATLAB Function/1(pseudoranges) -> Estimated Pseudoranges/1
  Predicted User States/1 -> Bus Selector3/1, Bus Selector/1
  MATLAB Function1/1(carrFrequency) -> Add/1, Estimated Carrier Frequencies/1
  Bus Selector/1 -> MATLAB Function/1(usrX)  "<x>"
  Bus Selector/2 -> MATLAB Function/2(usrY)  "<y>"
  Bus Selector/3 -> MATLAB Function/3(usrZ)  "<z>"
  Bus Selector/4 -> MATLAB Function/4(clk)  "<clk>"
  Satellite States/1 -> Bus Selector1/1, Bus Selector2/1
  Bus Selector1/3 -> MATLAB Function/7(satZ)  "<satZ>"
  Bus Selector1/2 -> MATLAB Function/6(satY)  "<satY>"
  Bus Selector1/1 -> MATLAB Function/5(satX)  "<satX>"
  MATLAB Function/2(unitVectors) -> MATLAB Function1/1(unitVectors)
  Bus Selector2/3 -> MATLAB Function1/7(satW)  "<satW>"
  Bus Selector2/2 -> MATLAB Function1/6(satV)  "<satV>"
  Bus Selector2/1 -> MATLAB Function1/5(satU)  "<satU>"
  Bus Selector3/3 -> MATLAB Function1/4(usrW)  "<w>"
  Bus Selector3/2 -> MATLAB Function1/3(usrV)  "<v>"
  Bus Selector3/1 -> MATLAB Function1/2(usrU)  "<u>"
  Add/1 -> Estimated Doppler/1
  Constant/1 -> Add/2
  Constant1/1 -> MATLAB Function1/8(clkDrift)
  Constant2/1 -> MATLAB Function1/9(L1Freq)
  Constant3/1 -> MATLAB Function1/10(IFFreq)
  Bus Selector2/4 -> Estimated SV Clock Bias/1  "<satClkCorr>"

== system DA40_Flight_Model/Correlator Simulation/Subsystem1/Subsystem2/Subsystem1 ==
  sampleVector : Inport
  carrierChangePerSample : Inport  Port=2
  measuredCarrierFrequency : Inport  Port=3
  codeChangePerSample : Inport  Port=4
  initialCodePhase : Inport  Port=5
  MATLAB Function1 : MATLAB Function  TreatAsAtomicUnit=on
  MATLAB Function3 : MATLAB Function  TreatAsAtomicUnit=on
  sampleVector1 : InportShadow
  MeasuredCarrierFrequency : Outport
  MeasuredCodeFrequency : Outport  Port=2
  wires:
  MATLAB Function3/1(MeasuredCarrierFrequency) -> MeasuredCarrierFrequency/1
  carrierChangePerSample/1 -> MATLAB Function3/2(carrierChangePerSample)
  measuredCarrierFrequency/1 -> MATLAB Function3/3(measuredCarrierFrequency)
  codeChangePerSample/1 -> MATLAB Function1/2(codeChangePerSample)
  initialCodePhase/1 -> MATLAB Function1/3(initialCodePhase)
  sampleVector/1 -> MATLAB Function3/1(sampleVector)
  MATLAB Function1/1(MeasuredCodeFrequency) -> MeasuredCodeFrequency/1
  sampleVector1/1 -> MATLAB Function1/1(sampleVector)

== system DA40_Flight_Model/Correlator Simulation/Subsystem1/Subsystem2/Subsystem2 ==
  initialCarrierFrequency : Inport
  initialDoppler : Inport  Port=2
  initialSVClockBias : Inport  Port=3
  estimatedCarrierFrequency : Inport  Port=4
  doppler : Inport  Port=5
  svClockBias : Inport  Port=6
  Constant : Constant  Value=1575.42e6
  Constant1 : Constant  Value=1.023e6
  Constant3 : Constant  Value=round((1/50)*16.368e6)
  Constant5 : Constant
  MATLAB Function1 : MATLAB Function  TreatAsAtomicUnit=on
  MATLAB Function2 : MATLAB Function  TreatAsAtomicUnit=on
  MATLAB Function3 : MATLAB Function  TreatAsAtomicUnit=on
  Subsystem2 : Subsystem
  sampleVector : Outport
  carrierChangePerSample : Outport  Port=2
  CarrierFrequency : Outport  Port=3
  codeChangePerSample : Outport  Port=4
  initialCodePhase : Outport  Port=5
  wires:
  Constant/1 -> MATLAB Function3/3(L1freq), MATLAB Function2/3(L1freq)
  Subsystem2/1(sampleVector) -> sampleVector/1
  Subsystem2/2(carrierChangePerSample) -> carrierChangePerSample/1
  Constant3/1 -> Subsystem2/1(samplesPerPDI)
  initialDoppler/1 -> MATLAB Function3/1(initialDoppler)
  Constant1/1 -> MATLAB Function3/2(initialChiprate), Subsystem2/7(chipRate), MATLAB Function2/2(chiprate)
  Subsystem2/5(initialCodePhase) -> initialCodePhase/1
  doppler/1 -> MATLAB Function2/1(doppler)
  Subsystem2/3(CarrierFrequency) -> CarrierFrequency/1
  initialSVClockBias/1 -> MATLAB Function1/2(initialSVClockBias)
  svClockBias/1 -> MATLAB Function1/1(svClockBias)
  MATLAB Function3/1(initialCodeFrequency) -> Subsystem2/4(initialCodeFrequency)
  MATLAB Function1/1(dSvClk) -> Subsystem2/8(dSvClk)
  estimatedCarrierFrequency/1 -> Subsystem2/3(measuredCarrierFrequency)
  Subsystem2/4(codeChangePerSample) -> codeChangePerSample/1
  initialCarrierFrequency/1 -> Subsystem2/2(initialCarrierFrequency)
  Constant5/1 -> Subsystem2/5("initialCodePhase ")
  MATLAB Function2/1(estimatedCodeFrequency) -> Subsystem2/6(measuredCodeFrequency)

== system DA40_Flight_Model/Correlator Simulation/Subsystem1/Subsystem2/Subsystem3 ==
  initialCarrierFrequency : Inport
  initialDoppler : Inport  Port=2
  initialSVClockBias : Inport  Port=3
  measuredCarrierFrequency : Inport  Port=4
  doppler : Inport  Port=5
  svClockBias : Inport  Port=6
  Constant : Constant  Value=1575.42e6
  Constant1 : Constant  Value=1.023e6
  Constant3 : Constant  Value=round((1/50)*16.368e6)
  Constant5 : Constant
  MATLAB Function1 : MATLAB Function  TreatAsAtomicUnit=on
  MATLAB Function2 : MATLAB Function  TreatAsAtomicUnit=on
  MATLAB Function3 : MATLAB Function  TreatAsAtomicUnit=on
  Subsystem2 : Subsystem
  sampleVector : Outport
  carrierChangePerSample : Outport  Port=2
  CarrierFrequency : Outport  Port=3
  codeChangePerSample : Outport  Port=4
  initialCodePhase : Outport  Port=5
  wires:
  MATLAB Function2/1(measuredCodeFrequency) -> Subsystem2/6(measuredCodeFrequency)
  Constant5/1 -> Subsystem2/5("initialCodePhase ")
  initialCarrierFrequency/1 -> Subsystem2/2(initialCarrierFrequency)
  Subsystem2/4(codeChangePerSample) -> codeChangePerSample/1
  measuredCarrierFrequency/1 -> Subsystem2/3(measuredCarrierFrequency)
  MATLAB Function1/1(dSvClk) -> Subsystem2/8(dSvClk)
  MATLAB Function3/1(initialCodeFrequency) -> Subsystem2/4(initialCodeFrequency)
  svClockBias/1 -> MATLAB Function1/1(svClockBias)
  initialSVClockBias/1 -> MATLAB Function1/2(initialSVClockBias)
  Subsystem2/3(CarrierFrequency) -> CarrierFrequency/1
  doppler/1 -> MATLAB Function2/1(doppler)
  Subsystem2/5(initialCodePhase) -> initialCodePhase/1
  Constant1/1 -> MATLAB Function2/2(chiprate), Subsystem2/7(chipRate), MATLAB Function3/2(initialChiprate)
  initialDoppler/1 -> MATLAB Function3/1(initialDoppler)
  Constant3/1 -> Subsystem2/1(samplesPerPDI)
  Subsystem2/2(carrierChangePerSample) -> carrierChangePerSample/1
  Subsystem2/1(sampleVector) -> sampleVector/1
  Constant/1 -> MATLAB Function2/3(L1freq), MATLAB Function3/3(L1freq)

== system DA40_Flight_Model/Correlator Simulation/Subsystem1/Subsystem2/Subsystem4 ==
  sampleVector : Inport
  carrierChangePerSample : Inport  Port=2
  measuredCarrierFrequency : Inport  Port=3
  codeChangePerSample : Inport  Port=4
  initialCodePhase : Inport  Port=5
  MATLAB Function1 : MATLAB Function  TreatAsAtomicUnit=on
  MATLAB Function3 : MATLAB Function  TreatAsAtomicUnit=on
  sampleVector1 : InportShadow
  EstimatedCarrierFrequency : Outport
  EstimatedCodeFrequency : Outport  Port=2
  wires:
  sampleVector1/1 -> MATLAB Function1/1(sampleVector)
  MATLAB Function1/1(MeasuredCodeFrequency) -> EstimatedCodeFrequency/1
  sampleVector/1 -> MATLAB Function3/1(sampleVector)
  initialCodePhase/1 -> MATLAB Function1/3(initialCodePhase)
  codeChangePerSample/1 -> MATLAB Function1/2(codeChangePerSample)
  measuredCarrierFrequency/1 -> MATLAB Function3/3(measuredCarrierFrequency)
  carrierChangePerSample/1 -> MATLAB Function3/2(carrierChangePerSample)
  MATLAB Function3/1(MeasuredCarrierFrequency) -> EstimatedCarrierFrequency/1

== system DA40_Flight_Model/Extended Kalman Filter/Noise Model/Navigation/DA-40 Equations of Motion ==
  Fb [lb] : Inport
  Mb [lb-ft] : Inport  Port=2
  Mass Properties : Inport  Port=3
  Bus Creator1 : BusCreator  Inputs=12
  Constant : Constant  Value=DCAM.FVDM.Vehicle.MassProp.r_cg
  Constant1 : Constant  Value=DCAM.FVDM.initialStates
  Constant4 : Constant  Value=DCAM.FVDM.Vehicle.MassProp.MOI  VectorParams1D=off
  Constant5 : Constant  Value=DCAM.FVDM.Vehicle.MassProp.InvMassMat
  Demux : Demux  Outputs=12
  Integrator2 : Integrator  InitialConditionSource=external
  MATLAB Function4 : MATLAB Function  TreatAsAtomicUnit=on
  States : Outport
  wires:
  Mb [lb-ft]/1 -> MATLAB Function4/4(M_B)
  Fb [lb]/1 -> MATLAB Function4/3(F_B)
  Mass Properties/1 -> MATLAB Function4/1(m)  "Mass"
  Constant4/1 -> MATLAB Function4/2(Ic_B)
  Constant1/1 -> Integrator2/2
  Integrator2/1 -> MATLAB Function4/5(X), Demux/1  "X-Vector"
  Constant/1 -> MATLAB Function4/6(CG)
  Constant5/1 -> MATLAB Function4/7(InvMassMatrix)
  Demux/1 -> Bus Creator1/1  "u"
  Demux/2 -> Bus Creator1/2  "v"
  Demux/3 -> Bus Creator1/3  "w"
  Demux/4 -> Bus Creator1/4  "p"
  Demux/5 -> Bus Creator1/5  "q"
  Demux/6 -> Bus Creator1/6  "r"
  Demux/7 -> Bus Creator1/7  "x"
  Demux/8 -> Bus Creator1/8  "y"
  Demux/9 -> Bus Creator1/9  "z"
  Demux/10 -> Bus Creator1/10  "phi"
  Demux/11 -> Bus Creator1/11  "theta"
  Demux/12 -> Bus Creator1/12  "psi"
  MATLAB Function4/1(X_Dot) -> Integrator2/1
  Bus Creator1/1 -> States/1
